simulink model "BOP"  (R2017b)
settings: Solver=ode15s  StartTime=0.0  StopTime=t_end  RelTol=1e-6
values from neighbouring files (symbols this model uses):
  Ib = [0.036 0 0; 0 0.036 0; 0 0 0.036]    [SimStarter.m]    (also in state_space.m = block.InputPort(4).Data)
  x_i = [r_ECI_i; v_ECI_i; q_i; w_i]    [SimStarter.m]
settings Model: Creator=mitchel1682  LastModifiedBy=mitchel1682

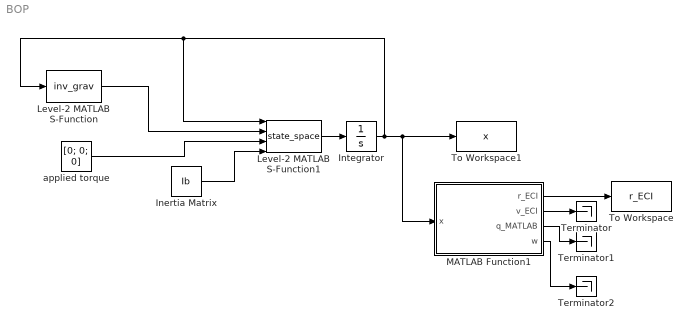
== system BOP ==
  "Inertia Matrix " : Constant  Value=Ib
  Integrator : Integrator  InitialCondition=x_i
  Level-2 MATLAB S-Function : M-S-Function  FunctionName=inv_grav
  Level-2 MATLAB S-Function1 : M-S-Function  FunctionName=state_space
  MATLAB Function1 : MATLAB Function  TreatAsAtomicUnit=on
  Terminator : Terminator
  Terminator1 : Terminator
  Terminator2 : Terminator
  To Workspace : ToWorkspace  VariableName=r_ECI  SampleTime=-1
  To Workspace1 : ToWorkspace  VariableName=x  SampleTime=-1
      settings: Save2DSignal=2-D array (concatenate along first dimension)
  "applied torque " : Constant  Value=[0; 0; 0]
  wires:
  "applied torque "/1 -> Level-2 MATLAB S-Function1/3
  Level-2 MATLAB S-Function/1 -> Level-2 MATLAB S-Function1/2
  "Inertia Matrix "/1 -> Level-2 MATLAB S-Function1/4
  Level-2 MATLAB S-Function1/1 -> Integrator/1
  Integrator/1 -> MATLAB Function1/1(x), To Workspace1/1, Level-2 MATLAB S-Function1/1, Level-2 MATLAB S-Function/1
  MATLAB Function1/1(r_ECI) -> To Workspace/1
  MATLAB Function1/3(q_MATLAB) -> Terminator1/1
  MATLAB Function1/2(v_ECI) -> Terminator/1
  MATLAB Function1/4(w) -> Terminator2/1

== matlab function BOP/MATLAB Function1 ==
  data: x input; r_ECI output; v_ECI output; q_MATLAB output; w output
function [r_ECI,v_ECI,q_MATLAB,w] = analysis_demux(x)

r_ECI = zeros(3,1);
r_ECI(1,1) = x(1,1);
r_ECI(2,1) = x(2,1);
r_ECI(3,1) = x(3,1);

v_ECI = zeros(3,1);
v_ECI(1,1) = x(4,1);
v_ECI(2,1) = x(5,1);
v_ECI(3,1) = x(6,1);

q_MATLAB = zeros(4,1); %output quaternion in MATLAB notation, not Dogan notation.
q_MATLAB(2,1) = x(7,1);
q_MATLAB(3,1) = x(8,1);
q_MATLAB(4,1) = x(9,1);
q_MATLAB(1,1) = x(10,1);

w = zeros(3,1);
w(1,1) = x(11,1);
w(2,1) = x(12,1);
w(3,1) = x(13,1);
end
